simulink model "Laboratoire2_R2011b"  (Simulink 7.8)
settings: Solver=FixedStepDiscrete  StartTime=0.0  StopTime=160  FixedStep=0.05  RelTol=1e-3
settings Model: Creator=plavoie  LastModifiedBy=plavoie
settings CodeAppCC: CustomSymbolStrType=$N$R$M_T
settings GRTTargetCC: CombineOutputUpdateFcns=on

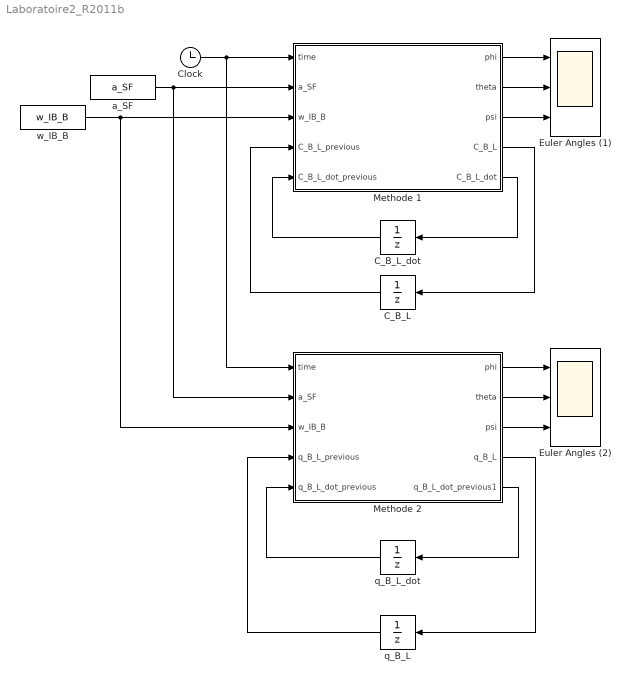
== system Laboratoire2_R2011b ==
  C_B_L : UnitDelay  X0=eye(3)  SampleTime=-1
  C_B_L_dot : UnitDelay  X0=zeros(3)  SampleTime=-1
  Clock : Clock
  Euler Angles (1) : Scope  NumInputPorts=3
      settings: YMin=-5~-5~-5  YMax=5~5~5
  Euler Angles (2) : Scope  NumInputPorts=3
      settings: YMin=-5~-5~-5  YMax=5~5~5
  Methode 1 : MATLAB Function  TreatAsAtomicUnit=on
      settings: PermitHierarchicalResolution=ParametersOnly
  Methode 2 : MATLAB Function  TreatAsAtomicUnit=on
      settings: PermitHierarchicalResolution=ParametersOnly
  a_SF : FromWorkspace  VariableName=a_SF  SampleTime=0
  q_B_L : UnitDelay  X0=[1;0;0;0]  SampleTime=-1
  q_B_L_dot : UnitDelay  X0=zeros(4,1)  SampleTime=-1
  w_IB_B : FromWorkspace  VariableName=w_IB_B  SampleTime=0
  wires:
  a_SF/1 -> Methode 1/2(a_SF), Methode 2/2(a_SF)
  w_IB_B/1 -> Methode 2/3(w_IB_B), Methode 1/3(w_IB_B)
  Methode 1/3(psi) -> Euler Angles (1)/3
  Methode 1/1(phi) -> Euler Angles (1)/1
  Methode 1/2(theta) -> Euler Angles (1)/2
  Methode 2/2(theta) -> Euler Angles (2)/2
  Methode 2/3(psi) -> Euler Angles (2)/3
  Methode 2/1(phi) -> Euler Angles (2)/1
  Clock/1 -> Methode 2/1(time), Methode 1/1(time)
  Methode 1/4(C_B_L) -> C_B_L/1
  C_B_L/1 -> Methode 1/4(C_B_L_previous)
  Methode 1/5(C_B_L_dot) -> C_B_L_dot/1
  C_B_L_dot/1 -> Methode 1/5(C_B_L_dot_previous)
  Methode 2/4(q_B_L) -> q_B_L/1
  q_B_L/1 -> Methode 2/4(q_B_L_previous)
  Methode 2/5(q_B_L_dot_previous1) -> q_B_L_dot/1
  q_B_L_dot/1 -> Methode 2/5(q_B_L_dot_previous)

== matlab function Methode 2 ==
  data: time input double; a_SF input double; phi output double; w_IB_B input double; theta output double; psi output double; q_B_L_previous input double; q_B_L_dot_previous input double; q_B_L output double; q_B_L_dot_previous1 output double
function [phi,theta,psi,q_B_L,q_B_L_dot_previous1] = fcn(time,a_SF,w_IB_B,q_B_L_previous,q_B_L_dot_previous)

%% Remplacez le code suivant par votre implémentation
theta = 0;
phi = 0;
psi = 0;
q_B_L = q_B_L_previous;
q_B_L_dot_previous = q_B_L_dot_previous;

== matlab function Methode 1 ==
  data: time input double; a_SF input double; phi output double; w_IB_B input double; theta output double; psi output double; a_SF_sum data_store_memory double; C_B_L output double; n data_store_memory double; C_B_L_dot output double; t data_store_memory double; C_B_L_previous input double; C_B_L_dot_previous input double
function [phi,theta,psi,C_B_L,C_B_L_dot] = fcn(time,a_SF,w_IB_B,C_B_L_previous,C_B_L_dot_previous)

%% Remplacez le code suivant par votre implémentation
theta = 0;
phi = 0;
psi = 0;
C_B_L = C_B_L_previous;
C_B_L_dot = C_B_L_dot_previous;
